simulink model "BF_realisation"  (R2021a)
settings: Solver=FixedStepAuto  StartTime=0.0  StopTime=inf  FixedStep=0.1  RelTol=1e-3  EnableMultiTasking=on
InitFcn:
  | Ts=0.1;
undefined symbols (not defined in the file): sigbuilder_block
libraries: simulink x2, arduinolib x2
settings Model: SimulationMode=external  SILPILModeSetting=veronly  ExtModeTrigDuration=2  Creator=PHAN DU  LastModifiedBy=anass
settings SolverCC: AlgebraicLoopSolver=TrustRegion  AutoInsertRateTranBlk=on
settings DataIOCC: ReturnWorkspaceOutputs=off
settings OptimizationCC: EnhancedBackFolding=on  PassReuseOutputArgsAs=Individual arguments  ZeroExternalMemoryAtStartup=off  ZeroInternalMemoryAtStartup=off  MaxStackSize=64  OptimizeBlockOrder=speed  DifferentSizesBufferReuse=on  EfficientTunableParamExpr=on
settings DebuggingCC: ParameterTunabilityLossMsg=error  SFMachineParentedDataDiag=warning
settings HardwareCC: ProdBitPerInt=16  ProdBitPerPointer=16  ProdBitPerSizeT=16  ProdBitPerPtrDiffT=16  ProdLargestAtomicFloat=None  ProdWordSize=8  ProdHWDeviceType=Atmel->AVR
settings SFSimCC: MATLABDynamicMemAlloc=off
settings RTWCC: SystemTargetFile=ert.tlc  HardwareBoard=Arduino Mega 2560  TemplateMakefile=ert_default_tmf  Toolchain=Arduino AVR  BuildConfiguration=Faster Runs
settings CodeAppCC: ForceParamTrailComments=on  IgnoreCustomStorageClasses=off  OperatorAnnotations=on  SimulinkDataObjDesc=on  SFDataObjDesc=on  InsertBlockDesc=on
settings ERTTargetCC: SupportContinuousTime=on  SupportVariableSizeSignals=on  ExtMode=on  ExtModeStaticAllocSize=2048  ExtModeMexArgs='127.0.0.1' 0 17725

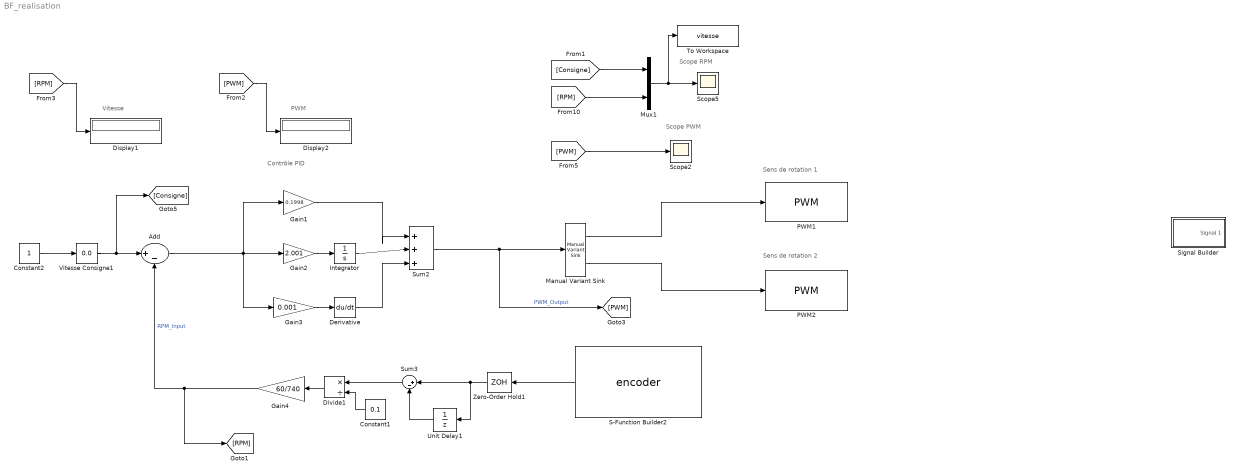
== system BF_realisation ==
  note: Scope PWM
  note: PWM
  note: Vitesse
  note: Contrôle PID
  note: Sens de rotation 1
  note: Sens de rotation 2
  note: Scope RPM
  Add : Sum  Inputs=|+-
  Constant1 : Constant  Value=0.1  SampleTime=0.1
  Constant2 : Constant
  Derivative : Derivative
  Display1 : Display
  Display2 : Display
  Divide1 : Product  Inputs=*/
  Gain1 : Gain  Gain=0.1998
  Gain2 : Gain  Gain=2.001
  Gain3 : Gain  Gain=0.001
  Gain4 : Gain  Gain=60/740
  Integrator : Integrator
  Manual Variant Sink : simulink/Signal Routing/Manual Variant Sink  NumChoices=2  LabelModeActiveChoice=V_1
  Mux1 : Mux  Inputs=2
  PWM1 : arduinolib/PWM  pinNumber=5  frequencyType=Default  desiredFrequency=490.2  achievableFrequency=2
  PWM2 : arduinolib/PWM  pinNumber=6  frequencyType=Default  desiredFrequency=490.2  achievableFrequency=2
  S-Function Builder2 : S-Function  InitFcn=try, set_param(gcb,'FunctionName','encoder'), end  FunctionName=encoder  Parameters=int8(0),int8(3),int8(2)  SFunctionModules=encoder_wrapper  SFunctionDeploymentMode=off  EnableBusSupport=off  mask(S-Function Builder){}
      mask help: Simulink:masks:SFunctionBuilder_MD
      mask init:
      | val = [[.9  0.75 0.75 1 1 .9 .9 1]',[1 1 0.75 0.75 .9 .9 1 .9]'];try , sys = get_param(gcb,'SfunBuilderFcnName');if isempty(sys), sys = get_param(gcb,'FunctionName'); end,catch, sys = get_param(gcb,'FunctionName'); end
      settings: CopyFcn=set_param(gcbh,'LinkStatus','none')  PreSaveFcn=try, set_param(gcb,'FunctionName','encoder'), end  OpenFcn=sfunctionwizard(gcbh)
      mask Display: plot(val(:,1),val(:,2)),disp(sys),port_label('output',1,'pos')
  Scope2 : Scope
  Scope5 : Scope
  Sum2 : Sum  Inputs=|+++
  Sum3 : Sum  Inputs=|+-
  To Workspace : ToWorkspace  VariableName=vitesse  SaveFormat=Timeseries  SampleTime=-1
  Unit Delay1 : UnitDelay  SampleTime=-1  HasFrameUpgradeWarning=on
  Vitesse Consigne1 : simulink/Math Operations/Slider Gain  gain=0.0  low=0  high=1000
  Zero-Order Hold1 : ZeroOrderHold  SampleTime=0.1
  Signal Builder : Subsystem  Tag=STV Subsys  IOType=siggen  LoadFcn=sigbuilder_block('load');  StartFcn=sigbuilder_block('start');  StopFcn=sigbuilder_block('stop');  ClipboardFcn=sigbuilder_block('clipboard');  mask(Sigbuilder block){tuvar=[0:10]}
      mask help: Sigbuilder GUI
      mask init:
      | if ~strcmp(get_param(bdroot(gcbh),'SimulationStatus'),'stopped') tuvar = sigbuilder_block('maskInit'); end
      settings: CopyFcn=sigbuilder_block('copy');  DeleteFcn=sigbuilder_block('delete');  ModelCloseFcn=sigbuilder_block('modelClose');  PreSaveFcn=sigbuilder_block('preSave');  PauseFcn=sigbuilder_block('pause');  ContinueFcn=sigbuilder_block('continue');  NameChangeFcn=sigbuilder_block('namechange');  OpenFcn=sigbuilder_block('open',[437.6 199.2 550.4 400 ]);  CloseFcn=sigbuilder_block('close');
      mask Display: plot(0, 0, 100, 100,[2, 2, 32, 32, 2], [68, 8, 8, 68, 68],[32, 2], [38, 38], [32, 19, 2],[53, 60, 44], [32, 17, 17, 2],[16, 16, 31, 31]);txt = getActiveGroup(gcbh);text(2, 100, txt,'verticalAlignment', 'top');
  wires:
  Divide1/1 -> Gain4/1
  Unit Delay1/1 -> Sum3/2
  Sum3/1 -> Divide1/1
  S-Function Builder2/1 -> Zero-Order Hold1/1
  Zero-Order Hold1/1 -> Sum3/1, Unit Delay1/1
  Constant1/1 -> Divide1/2
  [PWM] -> Display2/1
  [RPM] -> Display1/1
  Gain4/1 -> Add/2, [RPM]  "RPM_Input"
  Constant2/1 -> Vitesse Consigne1/1
  Gain3/1 -> Derivative/1
  Sum2/1 -> Manual Variant Sink/1, [PWM]  "PWM_Output"
  Integrator/1 -> Sum2/2
  Add/1 -> Gain3/1, Gain1/1, Gain2/1
  Derivative/1 -> Sum2/3
  Gain2/1 -> Integrator/1
  Gain1/1 -> Sum2/1
  [PWM] -> Scope2/1
  Manual Variant Sink/1 -> PWM1/1
  Manual Variant Sink/2 -> PWM2/1
  Vitesse Consigne1/1 -> [Consigne], Add/1
  Mux1/1 -> To Workspace/1, Scope5/1
  [Consigne] -> Mux1/1
  [RPM] -> Mux1/2

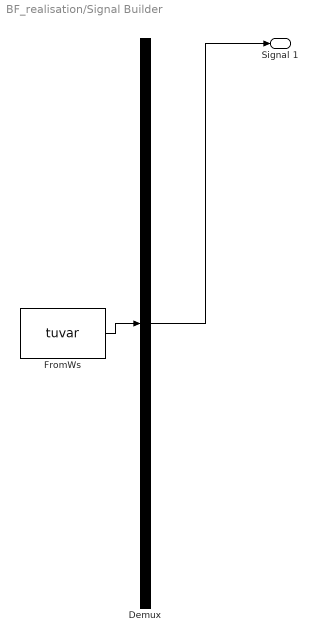
== system BF_realisation/Signal Builder ==
  Demux : Demux  Tag=STV Demux  Outputs=1
      settings: DisplayOption=none
  FromWs : FromWorkspace  Tag=STV FromWs  VariableName=tuvar
      SigBuilderData=|
      | common.afterFinalStr = 'Extrapolate'
      | common.sampleTime = 0
      | dataSet.timeRange = [0 10]
      | dataSet.name = 'Group 1'
      | sbobj.Groups.Name = 'Group 1'
      | sbobj.Groups.Signals.Name = 'Signal 1'
      | sbobj.Groups.Signals.XData = [0 4 4 6 6 10]
      | sbobj.Groups.Signals.YData = [0 0 1 1 0 0]
  Signal 1 : Outport  Tag=STV Outport
  wires:
  FromWs/1 -> Demux/1
  Demux/1 -> Signal 1/1
